simulink model "lab3bsim"  (R2023a)
settings: Solver=FixedStepAuto  StartTime=0.0  StopTime=1  FixedStep=1/1024  RelTol=1e-3
undefined symbols (not defined in the file or in its folder): lutdata, lutix
settings Model: Creator=a96an  LastModifiedBy=a96an
settings DataIOCC: ReturnWorkspaceOutputs=off

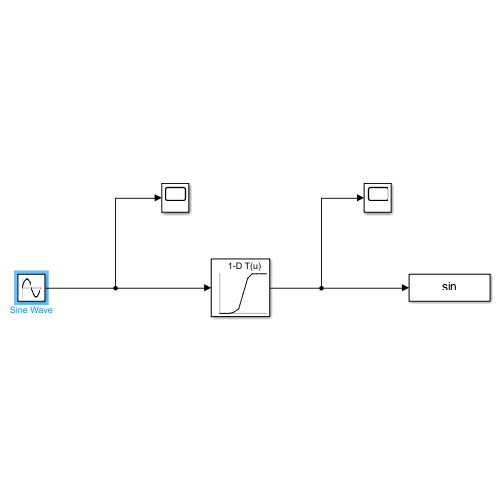
[thumbnail: Simulink's stored preview of the top-level diagram]
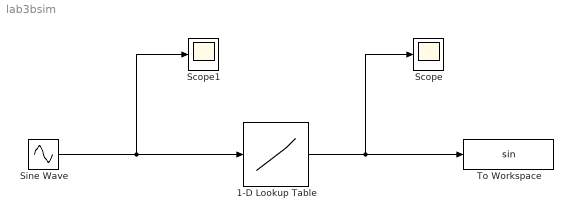
== system lab3bsim ==
  1-D Lookup Table : Lookup_n-D  NumberOfTableDimensions=1  BreakpointsForDimension1=lutix(2^10)  Table=lutdata(2^10)  InternalRulePriority=Speed  RndMeth=Simplest
  Scope : Scope
  Scope1 : Scope
  Sine Wave : Sin  Amplitude=1.5  Frequency=2*pi*5  SampleTime=0
  To Workspace : ToWorkspace  VariableName=sin  SaveFormat=Timeseries  SampleTime=-1
  wires:
  1-D Lookup Table/1 -> Scope/1, To Workspace/1
  Sine Wave/1 -> Scope1/1, 1-D Lookup Table/1
